simulink model "simulinksolution"  (R2024b)
settings: Solver=VariableStepAuto  StartTime=0.0  StopTime=20  RelTol=1e-3
undefined symbols (not defined in the file): C, L, R
settings Model: Creator=marti  LastModifiedBy=marti

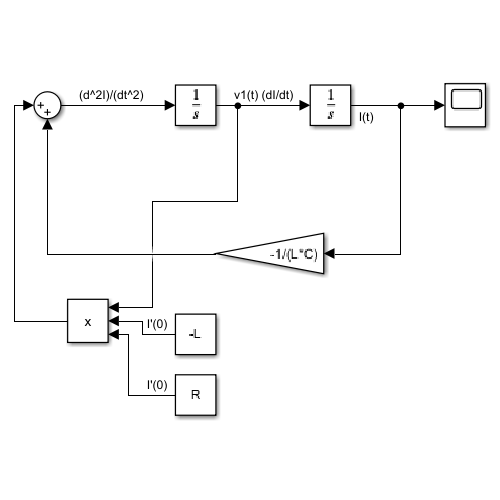
[thumbnail: Simulink's stored preview of the top-level diagram]
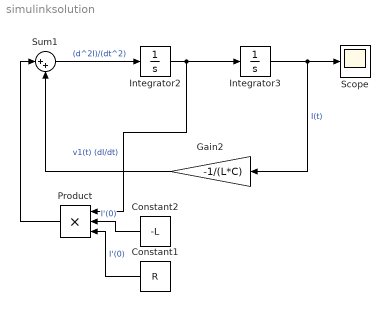
== system simulinksolution ==
  Constant1 : Constant  Value=R
  Constant2 : Constant  Value=-L
  Gain2 : Gain  Gain=-1/(L*C)
  Integrator2 : Integrator  InitialCondition=4
  Integrator3 : Integrator
  Product : Product  Inputs=3
  Scope : Scope
  Sum1 : Sum  Inputs=|++
  wires:
  Integrator2/1 -> Product/1, Integrator3/1  "v1(t) (dI/dt)"
  Sum1/1 -> Integrator2/1  "(d^2I)/(dt^2)"
  Integrator3/1 -> Gain2/1, Scope/1  "I(t)"
  Gain2/1 -> Sum1/2
  Constant2/1 -> Product/2  "I'(0)"
  Product/1 -> Sum1/1
  Constant1/1 -> Product/3  "I'(0)"
